simulink library "fdc"  (Simulink 8.1)
settings: Solver=ode45  StartTime=0.0  StopTime=10.0  RelTol=1e-3
undefined symbols (not defined in the file or in its folder): C_TICK_TIME_S, KJUD_FCWDeactVehSpeed_mps, KJUD_FCWVehAssignTimer_ms
libraries: hcu_lib x2, fva x1
settings Model: Creator=xsellart  LastModifiedBy=tescamilla

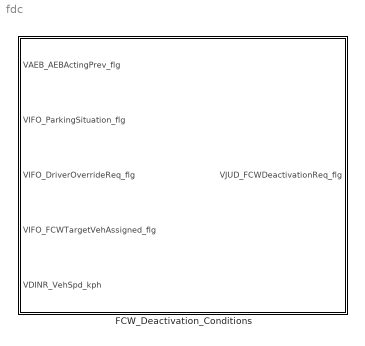
== system fdc ==
  FCW_Deactivation_Conditions : Subsystem

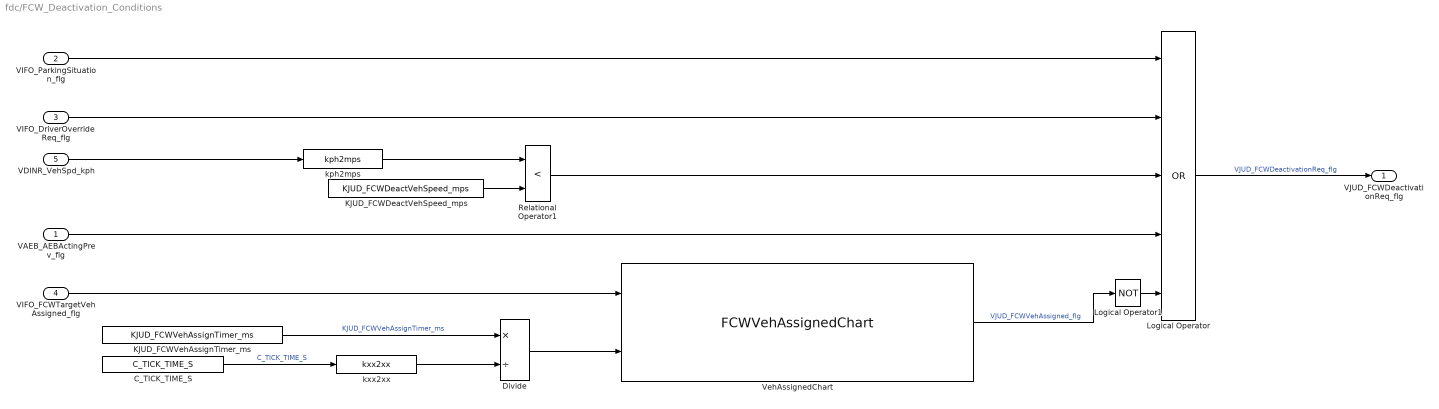
== system fdc/FCW_Deactivation_Conditions ==
  VAEB_AEBActingPrev_flg : Inport
  VIFO_ParkingSituation_flg : Inport  Port=2
  VIFO_DriverOverrideReq_flg : Inport  Port=3
  VIFO_FCWTargetVehAssigned_flg : Inport  Port=4
  VDINR_VehSpd_kph : Inport  Port=5
  C_TICK_TIME_S : Constant  Value=C_TICK_TIME_S
  Divide : Product  Inputs=*/
  KJUD_FCWDeactVehSpeed_mps : Constant  Value=KJUD_FCWDeactVehSpeed_mps  OutDataTypeStr=single
  KJUD_FCWVehAssignTimer_ms : Constant  Value=KJUD_FCWVehAssignTimer_ms  OutDataTypeStr=single
  Logical Operator : Logic  Operator=OR  Inputs=5  AllPortsSameDT=off  OutDataTypeStr=boolean
  Logical Operator1 : Logic  Operator=NOT  AllPortsSameDT=off  OutDataTypeStr=boolean
  Relational Operator1 : RelationalOperator  Operator=<  OutDataTypeStr=boolean
  VehAssignedChart : fva/FCWVehAssignedChart
  kph2mps : hcu_lib/kph2mps
  kxx2xx : hcu_lib/kxx2xx
  VJUD_FCWDeactivationReq_flg : Outport
  wires:
  Logical Operator/1 -> VJUD_FCWDeactivationReq_flg/1  "VJUD_FCWDeactivationReq_flg"
  Logical Operator1/1 -> Logical Operator/5
  VIFO_FCWTargetVehAssigned_flg/1 -> VehAssignedChart/1
  VAEB_AEBActingPrev_flg/1 -> Logical Operator/4
  Relational Operator1/1 -> Logical Operator/3
  KJUD_FCWDeactVehSpeed_mps/1 -> Relational Operator1/2
  VDINR_VehSpd_kph/1 -> kph2mps/1
  VIFO_DriverOverrideReq_flg/1 -> Logical Operator/2
  VIFO_ParkingSituation_flg/1 -> Logical Operator/1
  kph2mps/1 -> Relational Operator1/1
  Divide/1 -> VehAssignedChart/2
  C_TICK_TIME_S/1 -> kxx2xx/1  "C_TICK_TIME_S"
  kxx2xx/1 -> Divide/2
  KJUD_FCWVehAssignTimer_ms/1 -> Divide/1  "KJUD_FCWVehAssignTimer_ms"
  VehAssignedChart/1 -> Logical Operator1/1  "VJUD_FCWVehAssigned_flg"
